simulink subsystem "PieroControlado1mZ"  (R2023b)
settings: Solver=VariableStepAuto  StartTime=0.0  StopTime=10.0  RelTol=1e-3
undefined symbols (not defined in the file): DiscIntNeverNeededParam
settings Model: Creator=USUARIO  LastModifiedBy=USUARIO

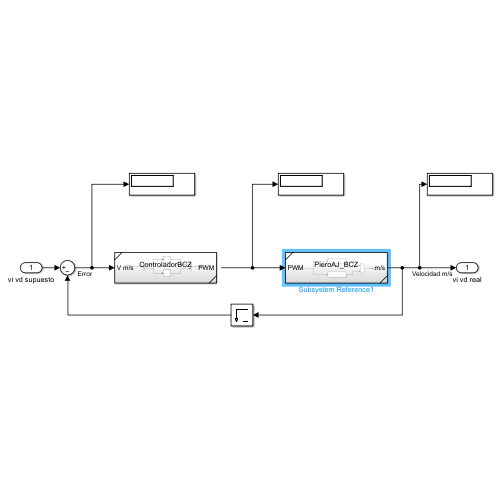
[thumbnail: Simulink's stored preview of the top-level diagram]
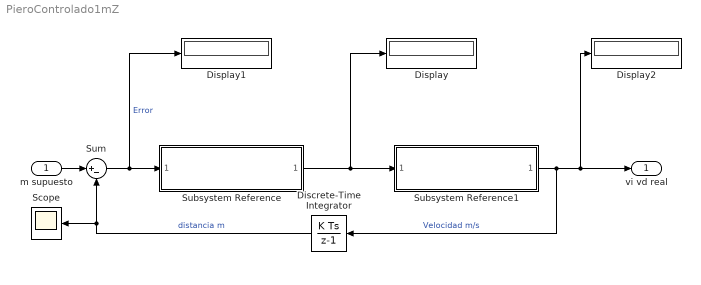
== system PieroControlado1mZ ==
  m supuesto : Inport
  Discrete-Time Integrator : DiscreteIntegrator  SampleTime=-1  ICPrevOutput=DiscIntNeverNeededParam  ICPrevScaledInput=DiscIntNeverNeededParam
  Display : Display
  Display1 : Display
  Display2 : Display
  Scope : Scope
  Subsystem Reference : Subsystem  ReferencedSubsystem=ControladorPos1mZ
  Subsystem Reference1 : Subsystem  ReferencedSubsystem=PieroAJ_BCZ
  Sum : Sum  Inputs=|+-
  vi vd real : Outport
  wires:
  Sum/1 -> Display1/1, Subsystem Reference/1  "Error"
  m supuesto/1 -> Sum/1
  Subsystem Reference/1 -> Display/1, Subsystem Reference1/1
  Subsystem Reference1/1 -> vi vd real/1, Display2/1, Discrete-Time Integrator/1  "Velocidad m/s"
  Discrete-Time Integrator/1 -> Scope/1, Sum/2  "distancia m"
